simulink model "symodel_simple_16a"  (R2016a)
settings: Solver=VariableStepAuto  StartTime=0.0  StopTime=10.0  RelTol=1e-3
libraries: simulink x1
settings Model: Creator=taehwan  LastModifiedBy=taehwan

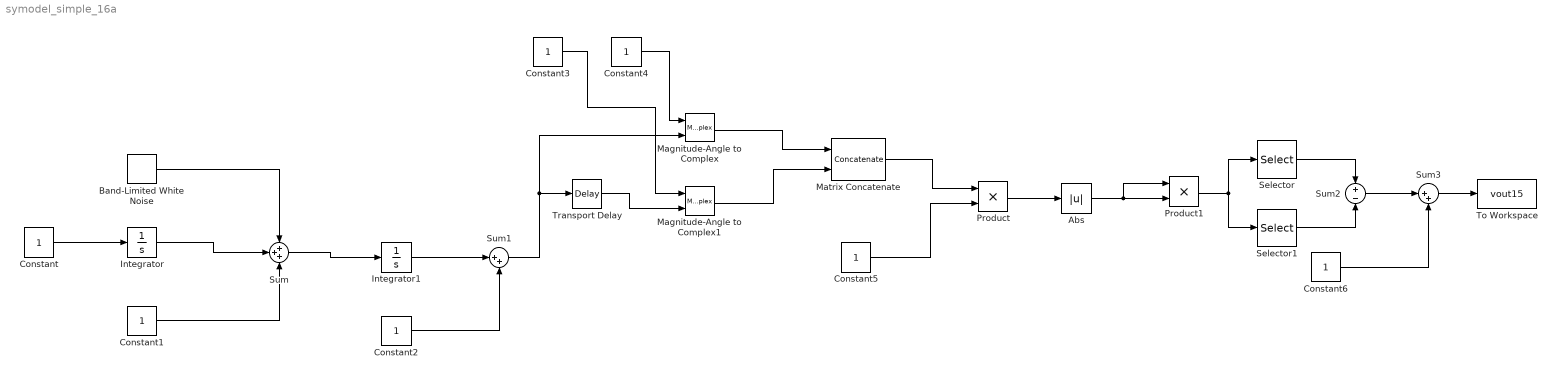
== system symodel_simple_16a ==
  Abs : Abs
  Band-Limited White Noise : simulink/Sources/Band-Limited White Noise  Cov=[0.1]  Ts=0.1  seed=[23341]
  Constant{,1..6} (7 alike) : Constant
  Integrator : Integrator
  Integrator1 : Integrator
  Magnitude-Angle to Complex : MagnitudeAngleToComplex
  Magnitude-Angle to Complex1 : MagnitudeAngleToComplex
  Matrix Concatenate : Concatenate  Mode=Multidimensional array  ConcatenateDimension=2
  Product : Product
  Product1 : Product
  Selector : Selector  InputPortWidth=3  IndexOptions=Index vector (dialog)  Indices=[1 3]  OutputSizes=1
  Selector1 : Selector  InputPortWidth=3  IndexOptions=Index vector (dialog)  Indices=[1 3]  OutputSizes=1
  Sum : Sum  Inputs=+++
  Sum1 : Sum  Inputs=|++
  Sum2 : Sum  Inputs=+|-
  Sum3 : Sum  Inputs=|++
  To Workspace : ToWorkspace  VariableName=vout15  SaveFormat=Timeseries  SampleTime=-1
  Transport Delay : TransportDelay
  wires:
  Sum1/1 -> Magnitude-Angle to Complex/2, Transport Delay/1
  Constant3/1 -> Magnitude-Angle to Complex1/1
  Transport Delay/1 -> Magnitude-Angle to Complex1/2
  Constant4/1 -> Magnitude-Angle to Complex/1
  Magnitude-Angle to Complex/1 -> Matrix Concatenate/1
  Magnitude-Angle to Complex1/1 -> Matrix Concatenate/2
  Integrator1/1 -> Sum1/1
  Constant2/1 -> Sum1/2
  Sum/1 -> Integrator1/1
  Integrator/1 -> Sum/2
  Constant1/1 -> Sum/3
  Band-Limited White Noise/1 -> Sum/1
  Constant/1 -> Integrator/1
  Matrix Concatenate/1 -> Product/1
  Constant5/1 -> Product/2
  Product/1 -> Abs/1
  Abs/1 -> Product1/1, Product1/2
  Product1/1 -> Selector1/1, Selector/1
  Selector/1 -> Sum2/1
  Selector1/1 -> Sum2/2
  Constant6/1 -> Sum3/2
  Sum2/1 -> Sum3/1
  Sum3/1 -> To Workspace/1
